simulink model "dc_motor"  (R2021a)
settings: Solver=VariableStepAuto  StartTime=0.0  StopTime=10.0  RelTol=1e-3
values from neighbouring files (symbols this model uses):
  bm = 0.018    [Data.m]    (also in uncertainty.m = ureal('bm', 0.018, 'percent', 20))
  Jw = J_motor + J_wheel    (= 0.0042488)    [Data.m]    (also in uncertainty.m = J_motor + J_wheel)
  Ke = 1.66e-2    (= 0.0166)    [Data.m]    (also in gear_test.m = gear*Kt; uncertainty.m = ureal('Ke', 1.66e-2, 'percent', 20))
  Kt = 1    [Data.m]    (also in gear_test.m = gear*0.876; uncertainty.m = ureal('Kt', 1, 'percent', 20))
  La = 3.2e-3    (= 0.0032)    [Data.m]    (also in uncertainty.m = ureal('La', 3.2e-3, 'percent', 20))
  Ra = 40.8    [Data.m]    (also in uncertainty.m = ureal('Ra', 40.8, 'percent', 20))
  V_nom = 24    [Data.m]    (also in uncertainty.m)
  x0 = [0.3 0 0 0]    [Data.m]
settings Model: Creator=jpss8  LastModifiedBy=jpss8

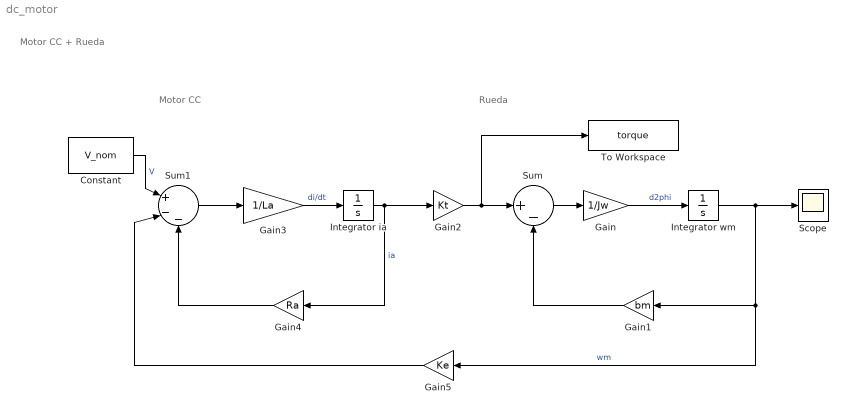
== system dc_motor ==
  note: Motor CC + Rueda
  note: Motor CC
  note: Rueda
  Constant : Constant  Value=V_nom
  Gain : Gain  Gain=1/Jw
  Gain1 : Gain  Gain=bm
  Gain2 : Gain  Gain=Kt
  Gain3 : Gain  Gain=1/La
  Gain4 : Gain  Gain=Ra
  Gain5 : Gain  Gain=Ke
  Integrator ia : Integrator  InitialCondition=x0(4)
  Integrator wm : Integrator  InitialCondition=x0(3)
  Scope : Scope
  Sum : Sum  Inputs=|+-
  Sum1 : Sum  Inputs=|+--
  To Workspace : ToWorkspace  VariableName=torque  SaveFormat=Structure With Time  SampleTime=-1
  wires:
  Gain5/1 -> Sum1/2
  Constant/1 -> Sum1/1  "V"
  Gain4/1 -> Sum1/3
  Sum1/1 -> Gain3/1
  Gain3/1 -> Integrator ia/1  "di/dt"
  Integrator ia/1 -> Gain4/1, Gain2/1  "ia"
  Gain2/1 -> To Workspace/1, Sum/1
  Gain1/1 -> Sum/2
  Integrator wm/1 -> Scope/1, Gain1/1, Gain5/1  "wm"
  Gain/1 -> Integrator wm/1  "d2phi"
  Sum/1 -> Gain/1
